simulink model "Funciones"  (R2024a)
settings: Solver=VariableStepAuto  StartTime=0.0  StopTime=10.0  RelTol=1e-3
settings Model: Creator=hmax6  LastModifiedBy=hmax6

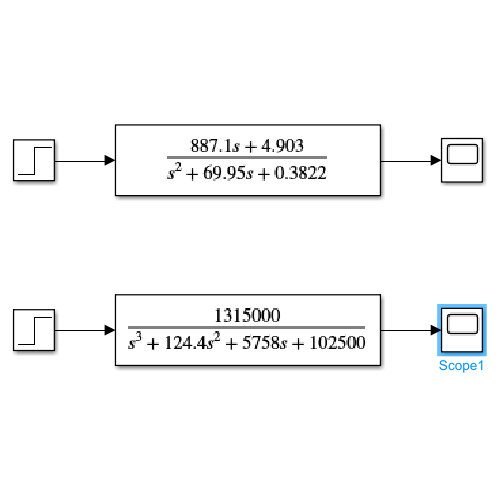
[thumbnail: Simulink's stored preview of the top-level diagram]
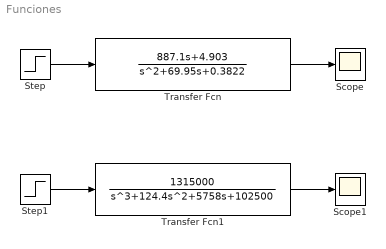
== system Funciones ==
  Scope : Scope
  Scope1 : Scope
  Step : Step  Time=0.05  After=12  SampleTime=0
  Step1 : Step  Time=0.05  After=12  SampleTime=0
  Transfer Fcn : TransferFcn  Numerator=[887.1 4.903]  Denominator=[1 69.95 0.3822]
  Transfer Fcn1 : TransferFcn  Numerator=[1315000]  Denominator=[1 124.4 5758 102500]
  wires:
  Step/1 -> Transfer Fcn/1
  Transfer Fcn/1 -> Scope/1
  Transfer Fcn1/1 -> Scope1/1
  Step1/1 -> Transfer Fcn1/1
